simulink model "Fuel_Cell_IV_Characteristic"  (R2021b)
settings: Solver=VariableStepAuto  StartTime=0.0  StopTime=Tsim  RelTol=1e-3
InitFcn:
  | V_init = 10;
values from neighbouring files (symbols this model uses):
  I_array = [0 40 80 120 160 200 230]    [script_execute.m]
  Ns = 48    [script_execute.m]
  qh2_supply = linspace(0, FuelCell.Max_Qfuel-FuelCell.Min_Qfuel, 5)    [script_execute.m]
  Tsim = 360    [script_execute.m]
  V_array = [46.6 38.7 36.6 34.7 32.7 31.0 29.5]    [script_execute.m]
undefined symbols (not defined in the file or in its folder): FuelCell
libraries: fl_lib x17, ee_lib x2, nesl_utility x2
settings Model: Creator=jsagardu  LastModifiedBy=jsagardu
settings SolverCC: AlgebraicLoopSolver=TrustRegion
settings DataIOCC: ReturnWorkspaceOutputs=off
settings DebuggingCC: SymbolicDimsDataTypeCodeGenerationDiagnostic=none  SFMachineParentedDataDiag=warning
settings SFSimCC: CustomCodeUndefinedFunction=UseInterfaceOnly
settings SimscapeCC: SimscapeLogType=local  SimscapeLogLimitData=off  SimscapeLogDataHistory=10000

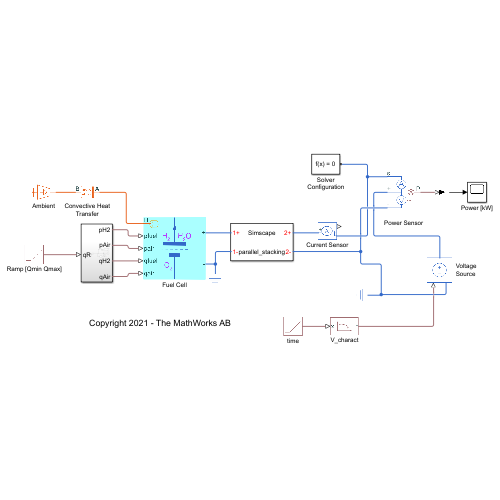
[thumbnail: Simulink's stored preview of the top-level diagram]
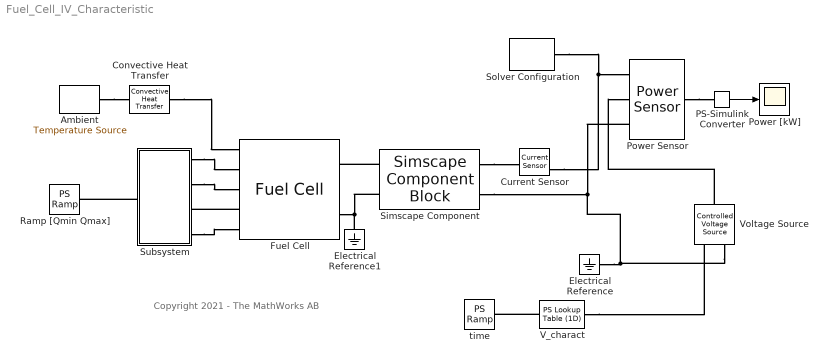
== system Fuel_Cell_IV_Characteristic ==
  note: Copyright 2021 - The MathWorks AB
  Ambient : fl_lib/Thermal/Thermal Sources/Temperature Source  temperature=293.15 K
  Convective Heat Transfer : fl_lib/Thermal/Thermal Elements/Convective Heat Transfer  area=120 cm^2  heat_tr_coeff=20 W/(m^2 * K)  T_specify=off  T_priority=None  T=0 K  T_nominal_specify=off  T_nominal_unit=K  T_nominal_value=1  Q_specify=off  Q_priority=None  Q=0 W  Q_nominal_specify=off  Q_nominal_unit=W  Q_nominal_value=1
  Current Sensor : fl_lib/Electrical/Electrical Sensors/Current Sensor
      settings: LogSimulationData=on
  Electrical Reference : fl_lib/Electrical/Electrical Elements/Electrical Reference
  Electrical Reference1 : fl_lib/Electrical/Electrical Elements/Electrical Reference
  Fuel Cell : ee_lib/Sources/Fuel Cell  model_fidelity=ee.enum.fuelcell.fidelity.detailed  Eoc=FuelCell.OpenCircuitVoltage V  A=FuelCell.TafelSlope V  ri=FuelCell.InternalResistance Ohm  i0=FuelCell.ExchangeCurrent A  i_lim=FuelCell.CollapseCurrent A  N_cell=Ncell  number_unit=Nu  pH2_nom=FuelCell.NomH2_Pressure Pa  pO2_nom=FuelCell.NomAir_Pressure Pa  xH2=FuelCell.Concentration(1)  xO2=FuelCell.Concentration(2)  xW=FuelCell.Concentration(3)  dyn=ee.enum.include.no  Rd=0.005 Ohm  tau=10 s  Tnom=293.15 K  thermal_mass=15000 J/K  iFC_specify=off  iFC_priority=High  iFC=10 A  iFC_nominal_specify=off  iFC_nominal_unit=A  iFC_nominal_value=1  vFC_specify=on  vFC_priority=High  vFC=FuelCell.InitVoltage V  vFC_nominal_specify=off  vFC_nominal_unit=V  vFC_nominal_value=1  temperature_specify=on  temperature_priority=High  temperature=293 K  temperature_nominal_specify=off  temperature_nominal_unit=K  temperature_nominal_value=1
      settings: SourceProductBaseCode=PS  LogSimulationData=on  InternalSimscapePortConfiguration="{\"Bottom\":[],\"Left\":[{\"id\":\"H\",\"label\":\"H\",\"type\":\"foundation.thermal.thermal\"},{\"id\":\"pfuel\",\"label\":\"pfuel\",\"type\":\"input\"},{\"id\":\"pair\",\"label\":\"pair\",\"type\":\"input\"},{\"id\":\"qfuel\",\"label\":\"qfuel\",\"type\":\"input\"},{\"id\":\"qair\",\"label\":\"qair\",\"type\":\"input\"}],\"Right\":[{\"id\":\"p\",\"label\":\"+\",\"type\":\"foundation.electrical.electrical\"},{\"id\":\"n\",\"label\":\"-\",\"type\":\"foundation.electrical.electrical\"}],\"Top\":[]}"
  PS-Simulink Converter : nesl_utility/PS-Simulink Converter  PhysicalDomain=network_engine_domain  SubClassName=ps_output  LeftPortType=input  RightPortType=output  PseudoPeriodic=off  Frequencies=[]  Unit=kW  AffineConversion=off
      settings: SourceProductName=Utilities
  Power Sensor : ee_lib/Sensors & Transducers/Power Sensor  measurement_type=1  averaging_period=1e-4 s
      settings: SourceProductBaseCode=PS  LogSimulationData=on
  Power [kW] : Scope
  Ramp [Qmin Qmax] : fl_lib/Physical Signals/Sources/PS Ramp  slope=(FuelCell.Max_Qfuel-FuelCell.Min_Qfuel)/360 lpm/s  start_time=Tstart s  initial_output=FuelCell.Init_Qfuel+FuelCell.Min_Qfuel lpm
      settings: SourceProductBaseCode=SS
  Simscape Component : SimscapeComponentBlock  SourceFile=parallel_stacking  ComponentPath=parallel_stacking  ComponentVariants="[\"parallel_stacking\"]"  ComponentVariantNames="[\"parallel_stacking\"]"  ClassName=parallel_stacking  SchemaVersion=1  n=Ns  R_vect=[.1, .005, .005] / Ns Ohm  i_vect=[min(I_array), 50, max(I_array)] A  i1_specify=off  i1_priority=None  i1=0 A  i1_nominal_specify=off  i1_nominal_unit=A  i1_nominal_value=1  v1_specify=off  v1_priority=None  v1=0 V  v1_nominal_specify=off  v1_nominal_unit=V  v1_nominal_value=1  i2_specify=off  i2_priority=None  i2=0 A  i2_nominal_specify=off  i2_nominal_unit=A  i2_nominal_value=1  v2_specify=off  v2_priority=None  v2=0 V  v2_nominal_specify=off  v2_nominal_unit=V  v2_nominal_value=1  R_specify=off  R_priority=None  R=0.01 Ohm  R_nominal_specify=off  R_nominal_unit=Ohm  R_nominal_value=1
      settings: CopyFcn=simscape.engine.sli.internal.componentblockcallback(gcbh,'COPY')  PreCopyFcn=simscape.engine.sli.internal.componentblockcallback(gcbh,'PRECOPY')  PreDeleteFcn=simscape.engine.sli.internal.componentblockcallback(gcbh,'PREDELETE')  InternalSimscapePortConfiguration="{\"Bottom\":[],\"Left\":[{\"id\":\"p1\",\"label\":\"1+\",\"type\":\"foundation.electrical.electrical\"},{\"id\":\"n1\",\"label\":\"1-\",\"type\":\"foundation.electrical.electrical\"}],\"Right\":[{\"id\":\"p2\",\"label\":\"2+\",\"type\":\"foundation.electrical.electrical\"},{\"id\":\"n2\",\"label\":\"2-\",\"type\":\"foundation.electrical.electrical\"}],\"Top\":[]}"
      mask Type: Transformer
  Solver Configuration : nesl_utility/Solver Configuration  PhysicalDomain=network_engine_domain  SubClassName=solver  LeftPortType=input  RightPortType=generic  Tones=[]  Harmonics=[]  SimulateNoise=off  Profile=off  UseLocalSampling=off  EnableSwitchedLinearOptims=on  FrequencyDomain=off  UseCCode=off  RelTol=0.001  AbsTol=1e-06  MinStep=1e-09  ToWorkspace=off  RevertToSquareIcSolve=off  NumHomotopyIterations=100  PhasorMode=off  PhasorModeNumHarmonics=1  DoDC=off  ResidualTolerance=1e-09  UseLocalSolver=off  LocalSolverChoice=NE_BACKWARD_EULER_ADVANCER  LocalSolverSampleTime=0.001  DoFixedCost=off  MaxNonlinIter=3  MaxModeIter=2  ComputeImpulses=off  ImpulseIterations=2  LinearAlgebra=auto  EquationFormulation=NE_TIME_EF  DelaysMemoryBudget=1024  AutomaticFiltering=on  FilteringTimeConstant=0.001  PartitionStorageMethod=AS_NEEDED  PartitionMemoryBudget=1024  PartitionMethod=ROBUST
      settings: SourceProductName=Utilities
  Subsystem : Subsystem
  V_charact : fl_lib/Physical Signals/Lookup Tables/PS Lookup Table (1D)  x=linspace(0,Tsim,numel(V_array)) s  f=V_array V  interp_method=simscape.enum.interpolation.smooth  extrap_method=simscape.enum.extrapolation.linear
      settings: SourceProductBaseCode=SS
  Voltage Source : fl_lib/Electrical/Electrical Sources/Controlled Voltage Source
      settings: LogSimulationData=on
  time : fl_lib/Physical Signals/Sources/PS Ramp  slope=1  start_time=0 s  initial_output=0 s
      settings: SourceProductBaseCode=SS
  wires:
  PS-Simulink Converter/1 -> Power [kW]/1
  connections:
  Fuel Cell/RConn2 -- Simscape Component/LConn2 -- Electrical Reference1/LConn1
  Solver Configuration/RConn1 -- Current Sensor/RConn2 -- Power Sensor/LConn1
  Voltage Source/LConn1 -- Power Sensor/LConn2
  Power Sensor/RConn1 -- PS-Simulink Converter/LConn1
  Convective Heat Transfer/LConn1 -- Fuel Cell/LConn1
  Ambient/LConn1 -- Convective Heat Transfer/RConn1
  Simscape Component/RConn1 -- Current Sensor/LConn1
  V_charact/LConn1 -- time/RConn1
  V_charact/RConn1 -- Voltage Source/RConn1
  Voltage Source/RConn2 -- Electrical Reference/LConn1 -- Simscape Component/RConn2 -- Power Sensor/LConn3
  Simscape Component/LConn1 -- Fuel Cell/RConn1
  Subsystem/RConn1 -- Fuel Cell/LConn2
  Subsystem/RConn2 -- Fuel Cell/LConn3
  Fuel Cell/LConn4 -- Subsystem/RConn3
  Subsystem/RConn4 -- Fuel Cell/LConn5
  Subsystem/LConn1 -- Ramp [Qmin Qmax]/RConn1

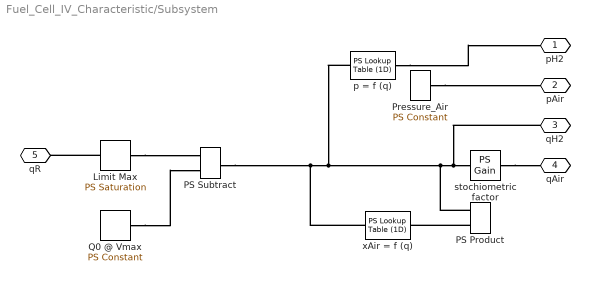
== system Fuel_Cell_IV_Characteristic/Subsystem ==
  Limit Max : fl_lib/Physical Signals/Nonlinear Operators/PS Saturation  upper_limit=(FuelCell.Max_Qfuel) lpm  lower_limit=(FuelCell.Min_Qfuel) lpm
      settings: SourceProductBaseCode=SS
  PS Product : fl_lib/Physical Signals/Functions/PS Product
  PS Subtract : fl_lib/Physical Signals/Functions/PS Subtract
  Pressure_Air : fl_lib/Physical Signals/Sources/PS Constant  constant=pAir bar
  Q0 @ Vmax : fl_lib/Physical Signals/Sources/PS Constant  constant=FuelCell.Min_Qfuel lpm
  p = f (q) : fl_lib/Physical Signals/Lookup Tables/PS Lookup Table (1D)  x=qh2_supply lpm  f=ph2_supply bar  interp_method=simscape.enum.interpolation.linear  extrap_method=simscape.enum.extrapolation.linear
      settings: SourceProductBaseCode=SS
  stochiometric factor : fl_lib/Physical Signals/Functions/PS Gain  gain=FuelCell.xAir
  xAir = f (q) : fl_lib/Physical Signals/Lookup Tables/PS Lookup Table (1D)  x=qh2_supply lpm  f=linspace(3.5,4.75,numel(qh2_supply))  interp_method=simscape.enum.interpolation.linear  extrap_method=simscape.enum.extrapolation.linear
      settings: SourceProductBaseCode=SS
  pH2 : PMIOPort  Side=Right
  pAir : PMIOPort  Port=2  Side=Right
  qH2 : PMIOPort  Port=3  Side=Right
  qAir : PMIOPort  Port=4  Side=Right
  qR : PMIOPort  Port=5  Side=Left
  connections:
  xAir = f (q)/LConn1 -- PS Subtract/RConn1 -- PS Product/LConn1 -- qH2/RConn1 -- stochiometric factor/LConn1 -- p = f (q)/LConn1
  Pressure_Air/RConn1 -- pAir/RConn1
  PS Product/LConn2 -- xAir = f (q)/RConn1
  p = f (q)/RConn1 -- pH2/RConn1
  stochiometric factor/RConn1 -- qAir/RConn1
  Q0 @ Vmax/RConn1 -- PS Subtract/LConn2
  Limit Max/LConn1 -- qR/RConn1
  Limit Max/RConn1 -- PS Subtract/LConn1
